simulink model "Gerador_de_dados_local"  (R2015a)
settings: Solver=ode45  StartTime=0.0  StopTime=1  RelTol=1e-3
settings Model: Creator=Afonso  LastModifiedBy=Élio

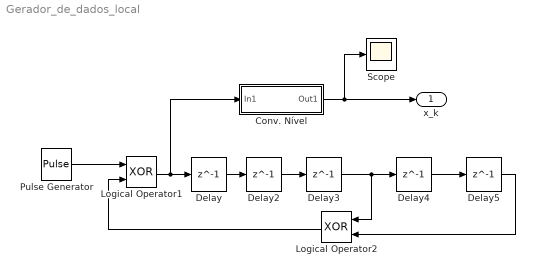
== system Gerador_de_dados_local ==
  Conv. Nível : Subsystem
  Delay : Delay  DelayLength=1  SampleTime=0.02
  Delay{2..5} (4 alike) : Delay  DelayLength=1
  Logical Operator1 : Logic  Operator=XOR  AllPortsSameDT=off  OutDataTypeStr=boolean
  Logical Operator2 : Logic  Operator=XOR  AllPortsSameDT=off  OutDataTypeStr=boolean
  Pulse Generator : DiscretePulseGenerator  PulseType=Time based  Amplitude=0  Period=0.02  PulseWidth=50
  Scope : Scope
  x_k : Outport
  wires:
  Delay2/1 -> Delay3/1
  Delay/1 -> Delay2/1
  Delay4/1 -> Delay5/1
  Delay3/1 -> Logical Operator2/1, Delay4/1
  Delay5/1 -> Logical Operator2/2
  Pulse Generator/1 -> Logical Operator1/1
  Logical Operator1/1 -> Conv. Nível/1(In1), Delay/1
  Logical Operator2/1 -> Logical Operator1/2
  Conv. Nível/1(Out1) -> x_k/1, Scope/1

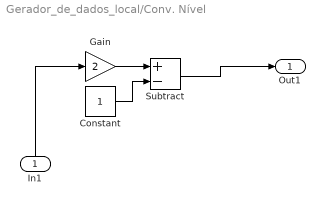
== system Gerador_de_dados_local/Conv. Nível ==
  In1 : Inport
  Constant : Constant
  Gain : Gain  Gain=2
  Subtract : Sum  Inputs=+-
  Out1 : Outport
  wires:
  In1/1 -> Gain/1
  Constant/1 -> Subtract/2
  Gain/1 -> Subtract/1
  Subtract/1 -> Out1/1
